simulink model "voltage_to_kelvin"  (R2020b)
settings: Solver=VariableStepAuto  StartTime=0.0  StopTime=10.0  RelTol=1e-3
libraries: simulink x1
settings Model: Creator=Milind  LastModifiedBy=Milind

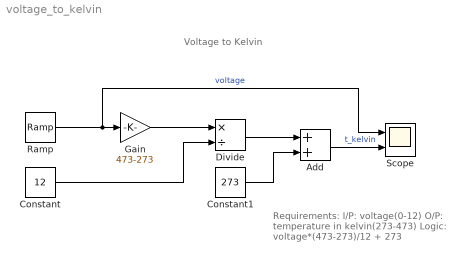
== system voltage_to_kelvin ==
  note: Requirements:
      | I/P: voltage(0-12)
      | O/P: temperature in kelvin(273-473)
      | Logic: voltage*(473-273)/12 + 273
  note: Voltage to Kelvin
  Add : Sum
  Constant : Constant  Value=12
  Constant1 : Constant  Value=273
  Divide : Product  Inputs=*/
  Gain : Gain  Gain=473-273
  Ramp : simulink/Sources/Ramp  slope=1  start=0  InitialOutput=0
  Scope : Scope  NumInputPorts=2
  wires:
  Ramp/1 -> Scope/1, Gain/1  "voltage"
  Gain/1 -> Divide/1
  Constant/1 -> Divide/2
  Divide/1 -> Add/1
  Constant1/1 -> Add/2
  Add/1 -> Scope/2  "t_kelvin"
